simulink model "Effect_of_AmbientTemp_on_Rint_Model"  (R2021a)
settings: Solver=VariableStepAuto  StartTime=0.0  StopTime=3600  FixedStep=1  RelTol=1e-3
values from neighbouring files (symbols this model uses):
  A_cell = cell_length*cell_width    (= 0.051302)    [Effect_of_AmbientTemp_RintModel.m]
  Capacity_LUT = [28.01,27.63,27.64]    [Effect_of_AmbientTemp_RintModel.m]
  Cp_cell = 810.5328    [Effect_of_AmbientTemp_RintModel.m]
  H_cell = 5    [Effect_of_AmbientTemp_RintModel.m]
  M_cell = 0.72    [Effect_of_AmbientTemp_RintModel.m]
  OCV_LUT = [3.49,3.51,3.52 ... (first row only)    [Effect_of_AmbientTemp_RintModel.m]
  R_int_LUT = [0.0117,0.0085,0.009 ... (first row only)    [Effect_of_AmbientTemp_RintModel.m]
  SOC_LUT = [0; 0.1; 0.25; 0.5; 0.75; 0.9; 1.0]    [Effect_of_AmbientTemp_RintModel.m]
  T_amb = 293.15    [Effect_of_AmbientTemp_RintModel.m]
  Temperature_LUT = [278.15,293.15,313.15]    [Effect_of_AmbientTemp_RintModel.m]
libraries: simulink x1
settings Model: Creator=gopin  LastModifiedBy=gopin

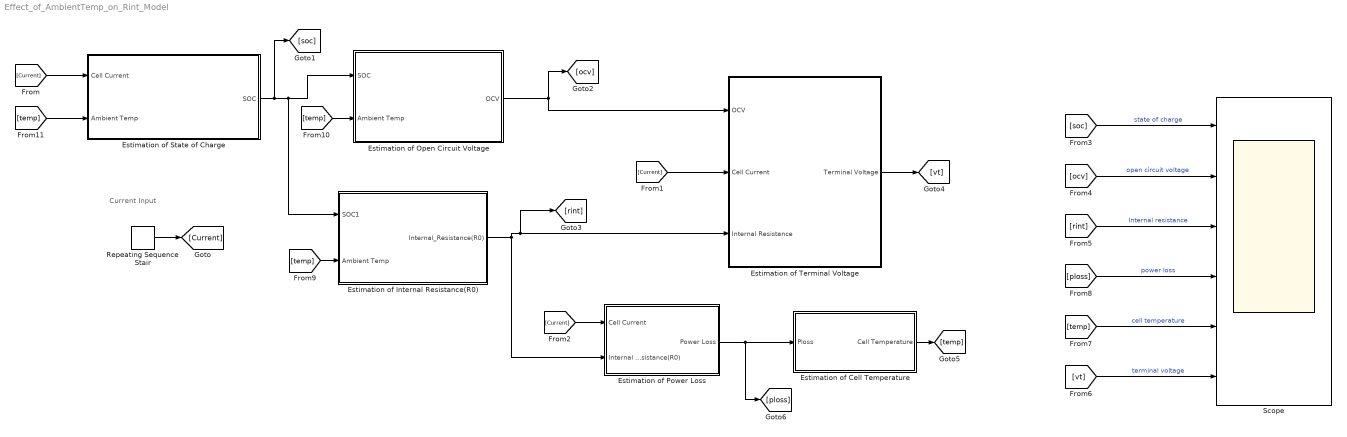
== system Effect_of_AmbientTemp_on_Rint_Model ==
  note: Current Input
  Estimation of Cell Temperature : Subsystem
  Estimation of Internal Resistance(R0) : Subsystem
  Estimation of Open Circuit Voltage : Subsystem
  Estimation of Power Loss : Subsystem
  "Estimation of State of Charge " : Subsystem
  Estimation of Terminal Voltage : Subsystem
  Repeating Sequence Stair : simulink/Sources/Repeating Sequence Stair  OutValues=[0 0 0 5 9 15 18 18 18 11 8 3 1]  tsamp=-1  OutMin=[]  OutMax=[]  OutDataTypeStr=double  OutputDataTypeScalingMode=double  OutDataType=fixdt(0,8)  ConRadixGroup=Best Precision: Vector-wise  OutScaling=2^-12
  Scope : Scope  NumInputPorts=6
  wires:
  [ploss] -> Scope/4  "power loss"
  Estimation of Internal Resistance(R0)/1(Internal_Resistance(R0)) -> [rint], Estimation of Terminal Voltage/3(Internal Resistance), Estimation of Power Loss/2(Internal Resistance(R0))
  [rint] -> Scope/3  "Internal resistance"
  [vt] -> Scope/6  "terminal voltage"
  Estimation of Power Loss/1(Power Loss) -> [ploss], Estimation of Cell Temperature/1(Ploss)
  Estimation of Terminal Voltage/1(Terminal Voltage) -> [vt]
  [Current] -> Estimation of Power Loss/1(Cell Current)
  [Current] -> Estimation of Terminal Voltage/2(Cell Current)
  [temp] -> Scope/5  "cell temperature"
  Estimation of Open Circuit Voltage/1(OCV) -> Estimation of Terminal Voltage/1(OCV), [ocv]
  [soc] -> Scope/1  "state of charge"
  Repeating Sequence Stair/1 -> [Current]
  [ocv] -> Scope/2  "open circuit voltage"
  Estimation of Cell Temperature/1(Cell Temperature) -> [temp]
  [Current] -> "Estimation of State of Charge "/1(Cell Current)
  "Estimation of State of Charge "/1(SOC) -> [soc], Estimation of Internal Resistance(R0)/1(SOC1), Estimation of Open Circuit Voltage/1(SOC)
  [temp] -> "Estimation of State of Charge "/2(Ambient Temp)
  [temp] -> Estimation of Internal Resistance(R0)/2(Ambient Temp)
  [temp] -> Estimation of Open Circuit Voltage/2(Ambient Temp)

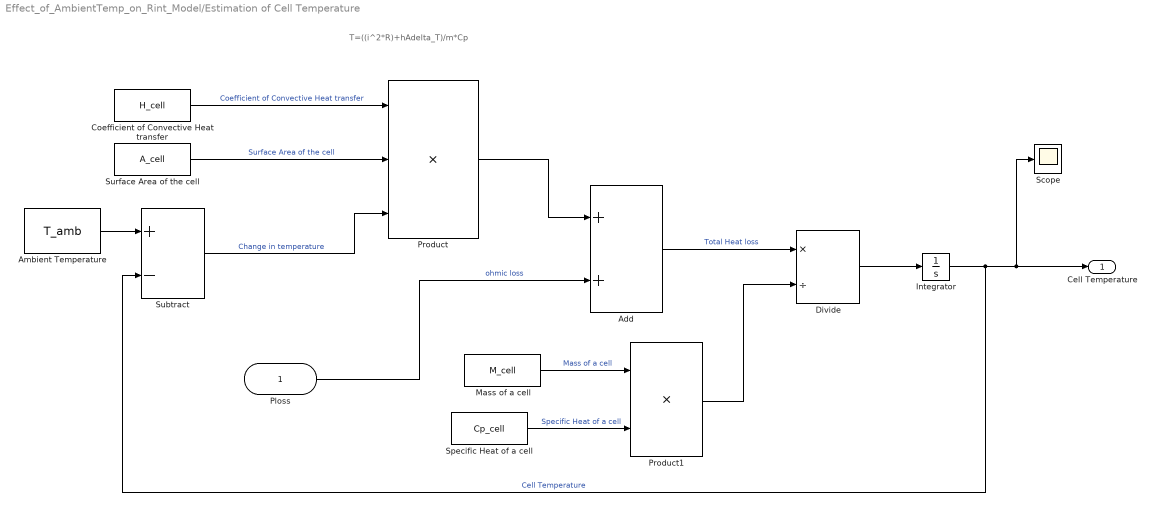
== system Effect_of_AmbientTemp_on_Rint_Model/Estimation of Cell Temperature ==
  note: T=((i^2*R)+hAdelta_T)/m*Cp
  Ploss : Inport
  Add : Sum
  Ambient Temperature : Constant  Value=T_amb
  Coefficient of Convective Heat transfer : Constant  Value=H_cell
  Divide : Product  Inputs=*/
  Integrator : Integrator  InitialCondition=T_amb  UpperSaturationLimit=353.15  LowerSaturationLimit=T_amb
  Mass of a cell : Constant  Value=M_cell
  Product : Product  Inputs=3
  Product1 : Product
  Scope : Scope
  Specific Heat of a cell : Constant  Value=Cp_cell
  Subtract : Sum  Inputs=+-
  Surface Area of the cell : Constant  Value=A_cell
  Cell Temperature : Outport
  wires:
  Ambient Temperature/1 -> Subtract/1
  Coefficient of Convective Heat transfer/1 -> Product/1  "Coefficient of Convective Heat transfer"
  Surface Area of the cell/1 -> Product/2  "Surface Area of the cell"
  Subtract/1 -> Product/3  "Change in temperature"
  Product/1 -> Add/1
  Ploss/1 -> Add/2  "ohmic loss"
  Add/1 -> Divide/1  "Total Heat loss"
  Product1/1 -> Divide/2
  Mass of a cell/1 -> Product1/1  "Mass of a cell"
  Specific Heat of a cell/1 -> Product1/2  "Specific Heat of a cell"
  Divide/1 -> Integrator/1
  Integrator/1 -> Subtract/2, Scope/1, Cell Temperature/1  "Cell Temperature"

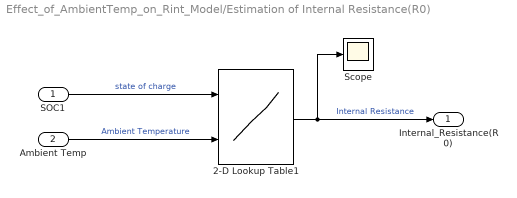
== system Effect_of_AmbientTemp_on_Rint_Model/Estimation of Internal Resistance(R0) ==
  SOC1 : Inport
  Ambient Temp : Inport  Port=2
  2-D Lookup Table1 : Lookup_n-D  BreakpointsForDimension1=SOC_LUT  BreakpointsForDimension2=Temperature_LUT  Table=R_int_LUT  InternalRulePriority=Speed  RndMeth=Simplest  InputSameDT=on
      settings: InputPortMap=u0,u1
  Scope : Scope
  Internal_Resistance(R0) : Outport
  wires:
  SOC1/1 -> 2-D Lookup Table1/1  "state of charge"
  2-D Lookup Table1/1 -> Scope/1, Internal_Resistance(R0)/1  "Internal Resistance"
  Ambient Temp/1 -> 2-D Lookup Table1/2  "Ambient Temperature"

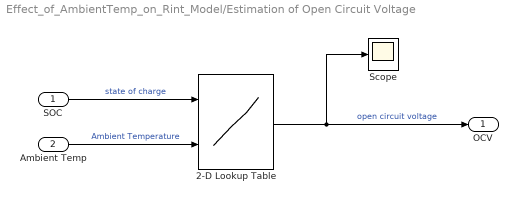
== system Effect_of_AmbientTemp_on_Rint_Model/Estimation of Open Circuit Voltage ==
  SOC : Inport
  Ambient Temp : Inport  Port=2
  2-D Lookup Table : Lookup_n-D  BreakpointsForDimension1=SOC_LUT  BreakpointsForDimension2=Temperature_LUT  Table=OCV_LUT  InternalRulePriority=Speed  RndMeth=Simplest  InputSameDT=on
      settings: InputPortMap=u0,u1
  Scope : Scope
  OCV : Outport
  wires:
  SOC/1 -> 2-D Lookup Table/1  "state of charge"
  2-D Lookup Table/1 -> Scope/1, OCV/1  "open circuit voltage"
  Ambient Temp/1 -> 2-D Lookup Table/2  "Ambient Temperature"

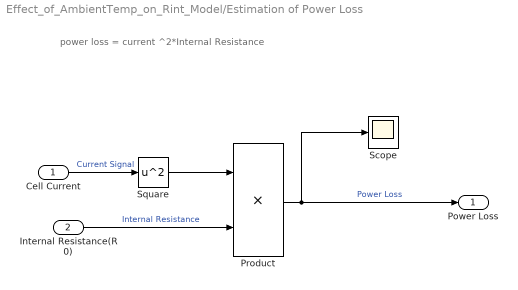
== system Effect_of_AmbientTemp_on_Rint_Model/Estimation of Power Loss ==
  note: power loss = current ^2*Internal Resistance
  Cell Current : Inport
  Internal Resistance(R0) : Inport  Port=2
  Product : Product
  Scope : Scope
  Square : Math  Operator=square  SaturateOnIntegerOverflow=on
  Power Loss : Outport
  wires:
  Cell Current/1 -> Square/1  "Current Signal"
  Square/1 -> Product/1
  Product/1 -> Scope/1, Power Loss/1  "Power Loss"
  Internal Resistance(R0)/1 -> Product/2  "Internal Resistance"

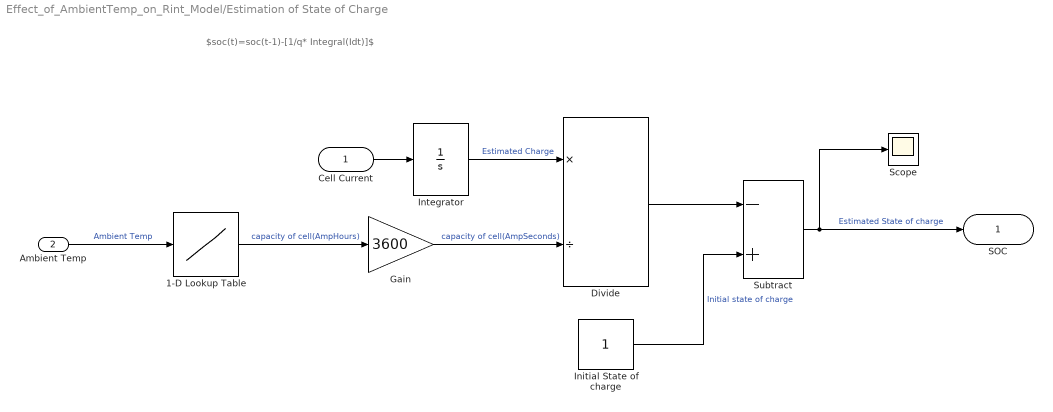
== system Effect_of_AmbientTemp_on_Rint_Model/Estimation of State of Charge  ==
  note: $soc(t)=soc(t-1)-[1/q* Integral(Idt)]$
  Cell Current : Inport
  Ambient Temp : Inport  Port=2
  1-D Lookup Table : Lookup_n-D  NumberOfTableDimensions=1  BreakpointsForDimension1=Temperature_LUT  Table=Capacity_LUT  InternalRulePriority=Speed  RndMeth=Simplest  InputSameDT=on
  Divide : Product  Inputs=*/
  Gain : Gain  Gain=3600
  Initial State of charge : Constant
  Integrator : Integrator
  Scope : Scope
  Subtract : Sum  Inputs=-+
  SOC : Outport
  wires:
  Initial State of charge/1 -> Subtract/2  "Initial state of charge"
  Subtract/1 -> Scope/1, SOC/1  "Estimated State of charge"
  Integrator/1 -> Divide/1  "Estimated Charge"
  Divide/1 -> Subtract/1
  Cell Current/1 -> Integrator/1
  1-D Lookup Table/1 -> Gain/1  "capacity of cell(AmpHours)"
  Gain/1 -> Divide/2  "capacity of cell(AmpSeconds)"
  Ambient Temp/1 -> 1-D Lookup Table/1  "Ambient Temp"

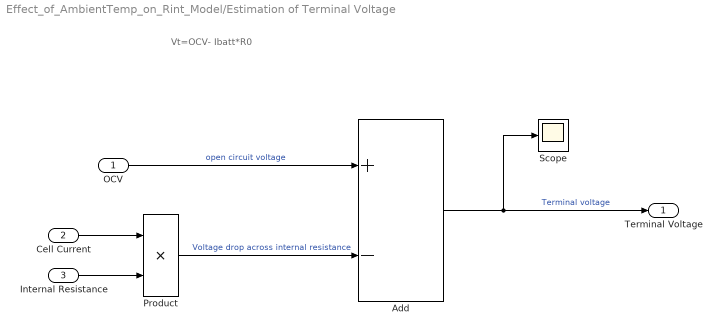
== system Effect_of_AmbientTemp_on_Rint_Model/Estimation of Terminal Voltage ==
  note: Vt=OCV- Ibatt*R0
  OCV : Inport
  Cell Current : Inport  Port=2
  Internal Resistance : Inport  Port=3
  Add : Sum  Inputs=+-
  Product : Product
  Scope : Scope
  Terminal Voltage : Outport
  wires:
  Add/1 -> Scope/1, Terminal Voltage/1  "Terminal voltage"
  OCV/1 -> Add/1  "open circuit voltage"
  Product/1 -> Add/2  "Voltage drop across internal resistance"
  Cell Current/1 -> Product/1
  Internal Resistance/1 -> Product/2
